simulink model "SimulacaoProjetoSala"  (R2023a)
settings: Solver=VariableStepAuto  StartTime=0.0  StopTime=2  RelTol=1e-3
values from neighbouring files (symbols this model uses):
  km = 30    [ProjetoSala1.m]
  tau = 100    [ProjetoSala1.m]
settings Model: Creator=a2270340  LastModifiedBy=a2270340

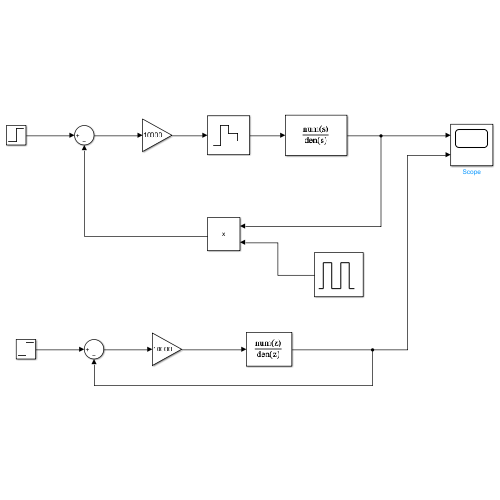
[thumbnail: Simulink's stored preview of the top-level diagram]
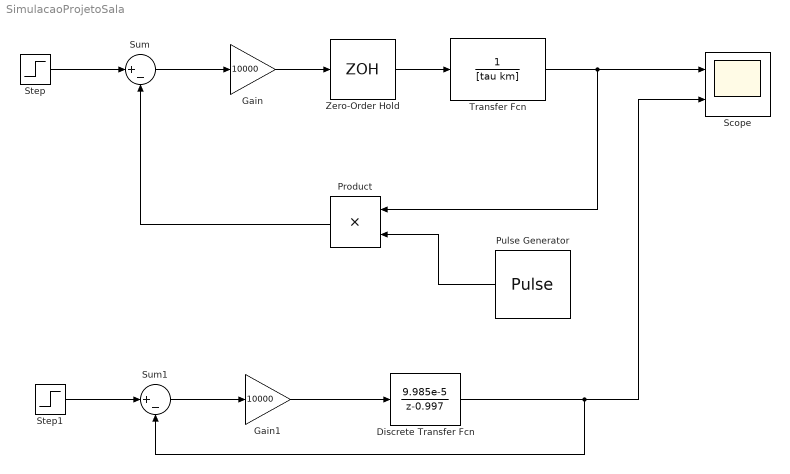
== system SimulacaoProjetoSala ==
  Discrete Transfer Fcn : DiscreteTransferFcn  Numerator=[9.985e-5]  Denominator=[1 -0.997]  SampleTime=0.01
  Gain : Gain  Gain=10000
  Gain1 : Gain  Gain=10000
  Product : Product
  Pulse Generator : DiscretePulseGenerator  PulseType=Time based  Period=0.01  PulseWidth=0.1
  Scope : Scope  NumInputPorts=2
  Step : Step  SampleTime=0
  Step1 : Step  SampleTime=0
  Sum : Sum  Inputs=|+-
  Sum1 : Sum  Inputs=|+-
  Transfer Fcn : TransferFcn  Denominator=[tau km]
  Zero-Order Hold : ZeroOrderHold  SampleTime=0.01
  wires:
  Sum/1 -> Gain/1
  Transfer Fcn/1 -> Product/1, Scope/1
  Step/1 -> Sum/1
  Gain/1 -> Zero-Order Hold/1
  Zero-Order Hold/1 -> Transfer Fcn/1
  Product/1 -> Sum/2
  Pulse Generator/1 -> Product/2
  Discrete Transfer Fcn/1 -> Scope/2, Sum1/2
  Step1/1 -> Sum1/1
  Sum1/1 -> Gain1/1
  Gain1/1 -> Discrete Transfer Fcn/1
